simulink model "Satellite_Design_Model_2019ver"  (R2019a)
settings: Solver=ode45  StartTime=0.0  StopTime=500  RelTol=1e-3
undefined symbols (not defined in the file or in its folder): km, s, sigbuilder_block
libraries: simulink_extras x10, sharedtransform x7, simulink x1, aerolibcelestial x1
settings Model: Creator=MSI  LastModifiedBy=MSI
settings SolverCC: ZeroCrossAlgorithm=Adaptive
settings OptimizationCC: LifeSpan=inf
settings DebuggingCC: IgnoredZcDiagnostic=none  SFExecutionAtInitializationDiag=none  ArithmeticOperatorsInVariantConditions=warning
settings HardwareCC: ProdBitPerSizeT=32  ProdBitPerPtrDiffT=32  ProdWordSize=32  ProdHWDeviceType=Specified
settings CodeAppCC: StateflowObjectComments=on

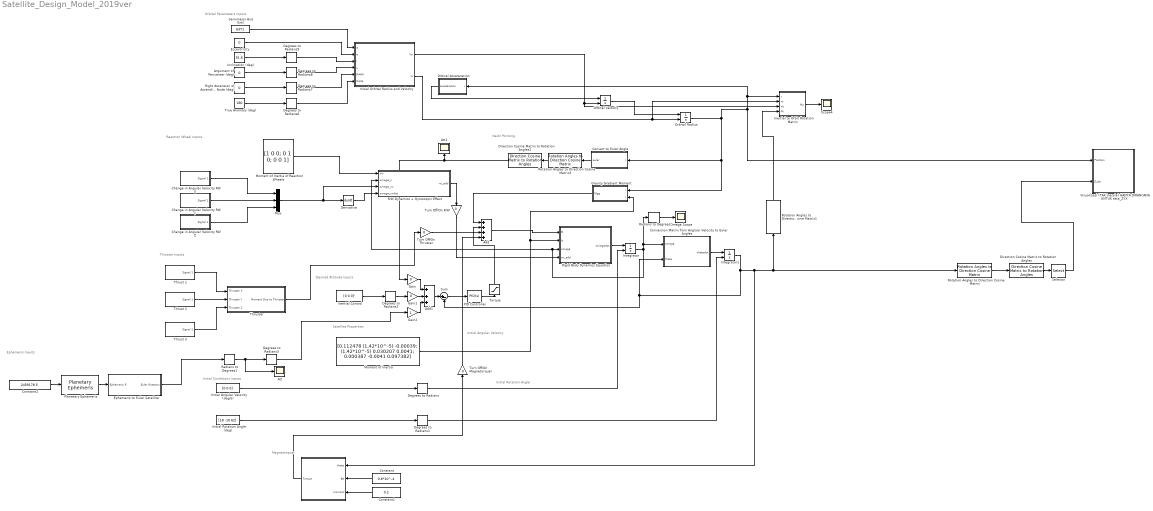
== system Satellite_Design_Model_2019ver ==
  note: Nadir Pointing
  note: Ephemeris Inputs
  note: Magnetorquer
  note: Initial Conditions Inputs
  note: Satellite Properties
  note: Desired Attitude Inputs
  note: Orbital Parameters Inputs
  note: Thruster Inputs
  note: Reaction Wheel Inputs
  note: Initial Rotation Angle
  note: Initial Angular Velocity
  " " : MATLAB Function  TreatAsAtomicUnit=on
  Add : Sum  Inputs=++++
  Add1 : Sum  Inputs=+++
  Argument of Pericenter (deg) : Constant  Value=0
  Att : Scope
  Att1 : Scope
  Change in Angular Velocity RW X : Subsystem  Tag=STV Subsys  LoadFcn=sigbuilder_block('load');  StartFcn=sigbuilder_block('start');  StopFcn=sigbuilder_block('stop');  ClipboardFcn=sigbuilder_block('clipboard');  mask(Sigbuilder block){tuvar=[0:10]}
      mask help: Simulink:masks:SigbuilderBlock_MD
      mask init:
      | if ~strcmp(get_param(bdroot(gcbh),'SimulationStatus'),'stopped') tuvar = sigbuilder_block('maskInit'); end
      settings: CopyFcn=sigbuilder_block('copy');  DeleteFcn=sigbuilder_block('delete');  ModelCloseFcn=sigbuilder_block('modelClose');  PreSaveFcn=sigbuilder_block('preSave');  PauseFcn=sigbuilder_block('pause');  ContinueFcn=sigbuilder_block('continue');  NameChangeFcn=sigbuilder_block('namechange');  OpenFcn=sigbuilder_block('open',[63.6 87.6 1024.8 449.4 ]);  CloseFcn=sigbuilder_block('close');
      mask Display: plot(0, 0, 100, 100,[2, 2, 32, 32, 2], [68, 8, 8, 68, 68],[32, 2], [38, 38], [32, 19, 2],[53, 60, 44], [32, 17, 17, 2],[16, 16, 31, 31]);txt = getActiveGroup(gcbh);text(2, 100, txt,'verticalAlignment', 'top');
  Change in Angular Velocity RW Y : Subsystem  Tag=STV Subsys  LoadFcn=sigbuilder_block('load');  StartFcn=sigbuilder_block('start');  StopFcn=sigbuilder_block('stop');  ClipboardFcn=sigbuilder_block('clipboard');  mask(Sigbuilder block){tuvar=[0:10]}
      mask help: Simulink:masks:SigbuilderBlock_MD
      mask init:
      | if ~strcmp(get_param(bdroot(gcbh),'SimulationStatus'),'stopped') tuvar = sigbuilder_block('maskInit'); end
      settings: CopyFcn=sigbuilder_block('copy');  DeleteFcn=sigbuilder_block('delete');  ModelCloseFcn=sigbuilder_block('modelClose');  PreSaveFcn=sigbuilder_block('preSave');  PauseFcn=sigbuilder_block('pause');  ContinueFcn=sigbuilder_block('continue');  NameChangeFcn=sigbuilder_block('namechange');  OpenFcn=sigbuilder_block('open',[0 30 1024.5 488.25 ]);  CloseFcn=sigbuilder_block('close');
      mask Display: plot(0, 0, 100, 100,[2, 2, 32, 32, 2], [68, 8, 8, 68, 68],[32, 2], [38, 38], [32, 19, 2],[53, 60, 44], [32, 17, 17, 2],[16, 16, 31, 31]);txt = getActiveGroup(gcbh);text(2, 100, txt,'verticalAlignment', 'top');
  Change in Angular Velocity RW Z : Subsystem  Tag=STV Subsys  LoadFcn=sigbuilder_block('load');  StartFcn=sigbuilder_block('start');  StopFcn=sigbuilder_block('stop');  ClipboardFcn=sigbuilder_block('clipboard');  mask(Sigbuilder block){tuvar=[0:10]}
      mask help: Simulink:masks:SigbuilderBlock_MD
      mask init:
      | if ~strcmp(get_param(bdroot(gcbh),'SimulationStatus'),'stopped') tuvar = sigbuilder_block('maskInit'); end
      settings: CopyFcn=sigbuilder_block('copy');  DeleteFcn=sigbuilder_block('delete');  ModelCloseFcn=sigbuilder_block('modelClose');  PreSaveFcn=sigbuilder_block('preSave');  PauseFcn=sigbuilder_block('pause');  ContinueFcn=sigbuilder_block('continue');  NameChangeFcn=sigbuilder_block('namechange');  OpenFcn=sigbuilder_block('open',[93.6 105.6 928.8 430.2 ]);  CloseFcn=sigbuilder_block('close');
      mask Display: plot(0, 0, 100, 100,[2, 2, 32, 32, 2], [68, 8, 8, 68, 68],[32, 2], [38, 38], [32, 19, 2],[53, 60, 44], [32, 17, 17, 2],[16, 16, 31, 31]);txt = getActiveGroup(gcbh);text(2, 100, txt,'verticalAlignment', 'top');
  Constant : Constant  Value=0.6*10^-4
  Constant1 : Constant  Value=0.2
  Constant2 : Constant  Value=2459178.5
  Conversion Matrix from Angluar Velocity to Euler Angles : MATLAB Function  TreatAsAtomicUnit=on
  Convert to Euler Angle : MATLAB Function  TreatAsAtomicUnit=on
  Degrees to Radians{,1..3,6..9} (8 alike) : simulink_extras/Transformations/Degrees to Radians
  Derivative : Derivative
  Direction Cosine Matrix to Rotation Angles : sharedtransform/Direction Cosine Matrix to Rotation Angles  rotationOrder=ZYX  aMode=aMode  action=None  tolerance=eps(2)
      settings: SourceProductBaseCode=AE,PW,MT,UV,VE,VP
  Direction Cosine Matrix to Rotation Angles2 : sharedtransform/Direction Cosine Matrix to Rotation Angles  rotationOrder=XYZ  aMode=aMode  action=None  tolerance=eps(2)
      settings: SourceProductName=Aerospace Blockset  SourceProductBaseCode=AE
  Eccentricity : Constant  Value=0
  Ephemeris to Euler Satellite : Subsystem
  Gain : Gain  Gain=0
  Gain1 : Gain  Gain=0
  Gain2 : Gain
  Gravity Gradient Moment : Subsystem
  Inclination (deg) : Constant  Value=51.6
  Inertial Control : Constant  Value=[0 0 0]'
  Inertial to Orbit Rotation Matrix : MATLAB Function  TreatAsAtomicUnit=on
  Initial Angular Velocity (deg/s) : Constant  Value=[0 0 0]
  Initial Orbital Radius and Velocity : MATLAB Function  TreatAsAtomicUnit=on
  Initial Rotation Angle (deg) : Constant  Value=[18 -10 62]
  Integrator : Integrator  InitialConditionSource=external
  Integrator1 : Integrator  InitialConditionSource=external
  Moment of Inertia : Constant  Value=[0.112478 (1.42*10^-5) -0.00039; (1.42*10^-5) 0.030207 0.0041; 0.000387 -0.0041 0.097382]
  Moment of Inertia of Reaction Wheels : Constant  Value=[1 0 0; 0 1 0; 0 0 1]
  Mux : Mux  Inputs=3
  Omega Scope : Scope
  Orbital Acceleration : MATLAB Function  TreatAsAtomicUnit=on
  Orbital Radius : Integrator  InitialConditionSource=external
  Orbital Velocity : Integrator  InitialConditionSource=external
  PID Controller : simulink/Continuous/PID Controller  Controller=PID  Form=Parallel  TimeDomain=Continuous-time  SampleTime=-1  IntegratorMethod=Forward Euler  FilterMethod=Forward Euler  ControllerParametersSource=internal  P=2  I=0  D=20  UseFilter=on  N=100  TunerSelectOption=Transfer Function Based (PID Tuner App)  InitialConditionSource=internal  InitialConditionForIntegrator=0  InitialConditionForFilter=0  DifferentiatorICPrevScaledInput=0  ExternalReset=none  TrackingMode=off  Kt=1  LimitOutput=off  UpperSaturationLimit=inf  LowerSaturationLimit=-inf  LinearizeAsGain=on  AntiWindupMode=none  Kb=1  POutMin=[]  POutMax=[]  IOutMin=[]  IOutMax=[]  DOutMin=[]  DOutMax=[]  NOutMin=[]  NOutMax=[]  SumOutMin=[]  SumOutMax=[]  SaturationOutMin=[]  SaturationOutMax=[]  PParamMin=[]  PParamMax=[]  IParamMin=[]  IParamMax=[]  DParamMin=[]  DParamMax=[]  NParamMin=[]  NParamMax=[]  KbParamMin=[]  KbParamMax=[]  KtParamMin=[]  KtParamMax=[]  KbOutMin=[]  KbOutMax=[]  KtOutMin=[]  KtOutMax=[]  IntegratorOutMin=[]  IntegratorOutMax=[]  FilterOutMin=[]  FilterOutMax=[]  SumI1OutMin=[]  SumI1OutMax=[]  SumI2OutMin=[]  SumI2OutMax=[]  SumI3OutMin=[]  SumI3OutMax=[]  SumI4OutMin=[]  SumI4OutMax=[]  SumDOutMin=[]  SumDOutMax=[]  DifferentiatorOutMin=[]  DifferentiatorOutMax=[]  FilterDiffOutCoefMin=[]  FilterDiffOutCoefMax=[]  ReciprocalOutMin=[]  ReciprocalOutMax=[]  SumDenOutMin=[]  SumDenOutMax=[]  SumNumOutMin=[]  SumNumOutMax=[]  DivideOutMin=[]  DivideOutMax=[]  IntegratorContinuousStateAttributes=''  IntegratorStateMustResolveToSignalObject=off  IntegratorRTWStateStorageClass=Auto  FilterContinuousStateAttributes=''  FilterStateMustResolveToSignalObject=off  FilterRTWStateStorageClass=Auto  ParallelPVariant=InternalParameters  IdealPVariant=Disabled  IVariant=InternalParameters  DVariant=InternalParameters  IntegratorVariant=Continuous  SatVariant=Disabled  AWVariant=Passthrough  PCopyVariant=Disabled  TRVariant=Disabled  FdbkBlocksVariant=Forward  IdealPFdbkVariant=Disabled  SatFdbkVariant=Disabled  DerivativeFilterVariant=ContFilter  NVariant=InternalParameters  NCopyVariant=Disabled  FilterICVariant=InternalICsFilter  IntegratorICVariant=InternalICs  ExternalResetVariant=Disabled  TRSumVariant=Passthrough  SumFdbkVariant=Disabled  SumVariant=Sum_PID
  Planetary Ephemeris : aerolibcelestial/Planetary Ephemeris  kmflag=km,km/s  epochflag=Julian date  de=DE405  nCenter=Earth  nTarget=Neptune  errorflag=Error  velflag=off
      settings: SourceProductName=Aerospace Blockset  SourceProductBaseCode=AE
  R/W Dynamics + Gyroscopic Effect : MATLAB Function  TreatAsAtomicUnit=on
  Radians to Degrees : simulink_extras/Transformations/Radians to Degrees
  Radians to Degrees1 : simulink_extras/Transformations/Radians to Degrees
  Right Ascension of Ascending Node (deg) : Constant  Value=0
  "Rigid Body Dynamics Equation " : MATLAB Function  TreatAsAtomicUnit=on
  Rotation Angles to Direction Cosine Matrix : sharedtransform/Rotation Angles to Direction Cosine Matrix  rotationOrder=XYZ  aMode=aMode
      settings: SourceProductBaseCode=AE,PW,MT,UV,VE,VP
  Rotation Angles to Direction Cosine Matrix1 : sharedtransform/Rotation Angles to Direction Cosine Matrix  rotationOrder=XYZ  aMode=aMode
      settings: SourceProductBaseCode=AE,PW,MT,UV,VE,VP
  Rotation Angles to Direction Cosine Matrix3 : sharedtransform/Rotation Angles to Direction Cosine Matrix  rotationOrder=ZYX  aMode=aMode
      settings: SourceProductBaseCode=AE
  Scope4 : Scope
  Selector : Selector  InputPortWidth=3  IndexOptions=Index vector (dialog)  Indices=[3 2 1]  OutputSizes=1
  Semimajor Axis (km) : Constant  Value=6371
  Sum : Sum  Inputs=|+-
  Thrust 1 : Subsystem  Tag=STV Subsys  LoadFcn=sigbuilder_block('load');  StartFcn=sigbuilder_block('start');  StopFcn=sigbuilder_block('stop');  ClipboardFcn=sigbuilder_block('clipboard');  mask(Sigbuilder block){tuvar=[0:10]}
      mask help: Simulink:masks:SigbuilderBlock_MD
      mask init:
      | if ~strcmp(get_param(bdroot(gcbh),'SimulationStatus'),'stopped') tuvar = sigbuilder_block('maskInit'); end
      settings: CopyFcn=sigbuilder_block('copy');  DeleteFcn=sigbuilder_block('delete');  ModelCloseFcn=sigbuilder_block('modelClose');  PreSaveFcn=sigbuilder_block('preSave');  PauseFcn=sigbuilder_block('pause');  ContinueFcn=sigbuilder_block('continue');  NameChangeFcn=sigbuilder_block('namechange');  OpenFcn=sigbuilder_block('open',[121.8 6 1024.8 449.4 ]);  CloseFcn=sigbuilder_block('close');
      mask Display: plot(0, 0, 100, 100,[2, 2, 32, 32, 2], [68, 8, 8, 68, 68],[32, 2], [38, 38], [32, 19, 2],[53, 60, 44], [32, 17, 17, 2],[16, 16, 31, 31]);txt = getActiveGroup(gcbh);text(2, 100, txt,'verticalAlignment', 'top');
  Thrust 2 : Subsystem  Tag=STV Subsys  LoadFcn=sigbuilder_block('load');  StartFcn=sigbuilder_block('start');  StopFcn=sigbuilder_block('stop');  ClipboardFcn=sigbuilder_block('clipboard');  mask(Sigbuilder block){tuvar=[0:10]}
      mask help: Simulink:masks:SigbuilderBlock_MD
      mask init:
      | if ~strcmp(get_param(bdroot(gcbh),'SimulationStatus'),'stopped') tuvar = sigbuilder_block('maskInit'); end
      settings: CopyFcn=sigbuilder_block('copy');  DeleteFcn=sigbuilder_block('delete');  ModelCloseFcn=sigbuilder_block('modelClose');  PreSaveFcn=sigbuilder_block('preSave');  PauseFcn=sigbuilder_block('pause');  ContinueFcn=sigbuilder_block('continue');  NameChangeFcn=sigbuilder_block('namechange');  OpenFcn=sigbuilder_block('open',[0 30 1024.5 488.25 ]);  CloseFcn=sigbuilder_block('close');
      mask Display: plot(0, 0, 100, 100,[2, 2, 32, 32, 2], [68, 8, 8, 68, 68],[32, 2], [38, 38], [32, 19, 2],[53, 60, 44], [32, 17, 17, 2],[16, 16, 31, 31]);txt = getActiveGroup(gcbh);text(2, 100, txt,'verticalAlignment', 'top');
  Thrust 3 : Subsystem  Tag=STV Subsys  LoadFcn=sigbuilder_block('load');  StartFcn=sigbuilder_block('start');  StopFcn=sigbuilder_block('stop');  ClipboardFcn=sigbuilder_block('clipboard');  mask(Sigbuilder block){tuvar=[0:10]}
      mask help: Simulink:masks:SigbuilderBlock_MD
      mask init:
      | if ~strcmp(get_param(bdroot(gcbh),'SimulationStatus'),'stopped') tuvar = sigbuilder_block('maskInit'); end
      settings: CopyFcn=sigbuilder_block('copy');  DeleteFcn=sigbuilder_block('delete');  ModelCloseFcn=sigbuilder_block('modelClose');  PreSaveFcn=sigbuilder_block('preSave');  PauseFcn=sigbuilder_block('pause');  ContinueFcn=sigbuilder_block('continue');  NameChangeFcn=sigbuilder_block('namechange');  OpenFcn=sigbuilder_block('open',[93.6 105.6 928.8 430.2 ]);  CloseFcn=sigbuilder_block('close');
      mask Display: plot(0, 0, 100, 100,[2, 2, 32, 32, 2], [68, 8, 8, 68, 68],[32, 2], [38, 38], [32, 19, 2],[53, 60, 44], [32, 17, 17, 2],[16, 16, 31, 31]);txt = getActiveGroup(gcbh);text(2, 100, txt,'verticalAlignment', 'top');
  Thruster : Subsystem
  Torque : Saturate  UpperLimit=0.00635  LowerLimit=-0.00635
  True Anomaly (deg) : Constant  Value=180
  Turn Off/On Magnetorquer : Gain  Gain=0
  Turn Off/On R/W : Gain  Gain=0
  Turn Off/On Thruster : Gain  Gain=0
  Visualisasi (TAK Inersia) HANYA DIRANCANG UNTUK teta_ZYX : Subsystem  mask(6DoF_Animation){u1=[-20000 20000 -20000 20000 -20000 20000], u2=1, u3=5000, u4=[0 0 0], u5=Fixed Position, u6=[40000 20000 30000], u7=30, u8=on}
      mask prompts: u1 "Axes limits [xmin xmax ymin ymax zmin zmax]:"; u2 "Time interval between updates:"; u3 "Size of craft displayed:"; u4 "Static object position [xp yp zp]:"; u5 "Enter view:"; u6 "Position of camera [xc yc zc]:"; u7 "View angle:"; u8 "Enable animation"
      mask init:
      | Config.axes = u1;
      | Config.update = u2;
      | Config.craft = u3;
      | Config.target = u4;
      | Config.camera_view = u5;
      | Config.camera_pos = u6;
      | Config.view = u7;
      | Config.Animenable = u8;
      | Config.Model = bdroot(gcb);
      mask TypeOptions u5: Fixed Position | Cockpit | Fly alongside
      mask Display:
      | port_label('input',1,'x_e','texmode','on');
      | port_label('input',2,'\phi \theta \psi','texmode','on');
      | [xp yp] = aeroimage('anim',gcbh);
      | patch(xp,yp)
  wires:
  Selector/1 -> Visualisasi (TAK Inersia) HANYA DIRANCANG UNTUK teta_ZYX/2(Euler)
  Direction Cosine Matrix to Rotation Angles/1 -> Selector/1
  Rotation Angles to Direction Cosine Matrix/1 -> Direction Cosine Matrix to Rotation Angles/1
  Integrator/1 -> Radians to Degrees/1, Conversion Matrix from Angluar Velocity to Euler Angles/1(omega), R/W Dynamics + Gyroscopic Effect/2(omega_s), "Rigid Body Dynamics Equation "/3(omega)
  Conversion Matrix from Angluar Velocity to Euler Angles/1(thetadot) -> Integrator1/1
  Degrees to Radians/1 -> Integrator/2
  Degrees to Radians1/1 -> Integrator1/2
  Initial Angular Velocity (deg/s)/1 -> Degrees to Radians/1
  Integrator1/1 -> Sum/2, Conversion Matrix from Angluar Velocity to Euler Angles/2(theta), Rotation Angles to Direction Cosine Matrix/1, Rotation Angles to Direction Cosine Matrix1/1, " "/1(theta)
  Radians to Degrees/1 -> Omega Scope/1
  Moment of Inertia/1 -> Gravity Gradient Moment/2(I), "Rigid Body Dynamics Equation "/2(Is)
  Degrees to Radians9/1 -> Initial Orbital Radius and Velocity/3(i)
  Eccentricity/1 -> Initial Orbital Radius and Velocity/2(e)
  Inertial to Orbit Rotation Matrix/1(Mo) -> Scope4/1
  Rotation Angles to Direction Cosine Matrix1/1 -> Inertial to Orbit Rotation Matrix/4(Mi)
  Initial Orbital Radius and Velocity/1(Vo) -> Inertial to Orbit Rotation Matrix/3(Vo), Orbital Velocity/2
  Degrees to Radians6/1 -> Initial Orbital Radius and Velocity/6(theta)
  Degrees to Radians8/1 -> Initial Orbital Radius and Velocity/4(u)
  Degrees to Radians7/1 -> Initial Orbital Radius and Velocity/5(RAAN)
  Initial Orbital Radius and Velocity/2(ro) -> Inertial to Orbit Rotation Matrix/2(ro), Orbital Radius/2
  Argument of Pericenter (deg)/1 -> Degrees to Radians8/1
  Right Ascension of Ascending Node (deg)/1 -> Degrees to Radians7/1
  Orbital Acceleration/1(acceleration) -> Orbital Velocity/1
  Inclination (deg)/1 -> Degrees to Radians9/1
  Orbital Velocity/1 -> Orbital Radius/1
  Semimajor Axis (km)/1 -> Initial Orbital Radius and Velocity/1(a)
  True Anomaly (deg)/1 -> Degrees to Radians6/1
  Thrust 1/1(Signal 1) -> Thruster/1(Thruster X)
  Thrust 2/1(Signal 1) -> Thruster/2(Thruster Y)
  Thrust 3/1(Signal 1) -> Thruster/3(Thruster Z)
  Gravity Gradient Moment/1(Mgg) -> Add/1
  Sum/1 -> PID Controller/1
  PID Controller/1 -> Torque/1
  Add/1 -> "Rigid Body Dynamics Equation "/1(M)
  Torque/1 -> Add/2
  Thruster/1(Moment Due to Thruster) -> Turn Off/On Thruster/1
  Change in Angular Velocity RW X/1(Signal 1) -> Mux/1
  Change in Angular Velocity RW Y/1(Signal 1) -> Mux/2
  Change in Angular Velocity RW Z/1(Signal 1) -> Mux/3
  "Rigid Body Dynamics Equation "/1(omegadot) -> Integrator/1
  Moment of Inertia of Reaction Wheels/1 -> R/W Dynamics + Gyroscopic Effect/1(Irw)
  Mux/1 -> Derivative/1, R/W Dynamics + Gyroscopic Effect/3(omega_rw)
  Derivative/1 -> R/W Dynamics + Gyroscopic Effect/4(omega_rwdot)
  R/W Dynamics + Gyroscopic Effect/1(rw_add) -> Turn Off/On R/W/1
  Turn Off/On R/W/1 -> "Rigid Body Dynamics Equation "/4(rw_add)
  Constant/1 -> " "/2(Be)
  Constant1/1 -> " "/3(moment)
  " "/1(Torque) -> Turn Off/On Magnetorquer/1
  Turn Off/On Magnetorquer/1 -> Add/4
  Turn Off/On Thruster/1 -> Add/3
  Inertial Control/1 -> Degrees to Radians2/1
  Constant2/1 -> Planetary Ephemeris/1
  Orbital Radius/1 -> Gravity Gradient Moment/1(r), Convert to Euler Angle/1(r), Visualisasi (TAK Inersia) HANYA DIRANCANG UNTUK teta_ZYX/1(Position), Inertial to Orbit Rotation Matrix/1(r), Orbital Acceleration/1(r)
  Rotation Angles to Direction Cosine Matrix3/1 -> Direction Cosine Matrix to Rotation Angles2/1
  Convert to Euler Angle/1(euler) -> Rotation Angles to Direction Cosine Matrix3/1
  Direction Cosine Matrix to Rotation Angles2/1 -> Att1/1, Gain/1
  Planetary Ephemeris/1 -> Ephemeris to Euler Satellite/1(Ephemeris R)
  Add1/1 -> Sum/1
  Degrees to Radians2/1 -> Gain1/1
  Gain/1 -> Add1/1
  Gain1/1 -> Add1/2
  Gain2/1 -> Add1/3
  Ephemeris to Euler Satellite/1(Euler Rotation) -> Radians to Degrees1/1
  Initial Rotation Angle (deg)/1 -> Degrees to Radians1/1
  Degrees to Radians3/1 -> Gain2/1
  Radians to Degrees1/1 -> Att/1, Degrees to Radians3/1

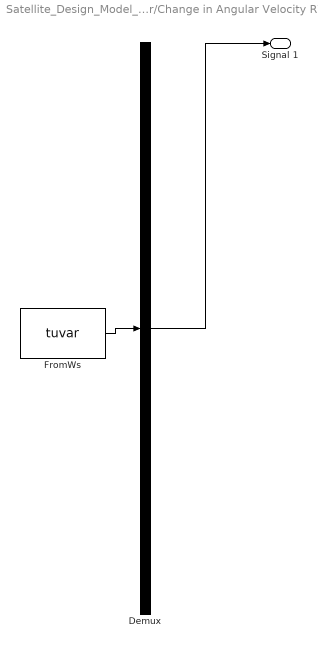
== system Satellite_Design_Model_2019ver/Change in Angular Velocity RW X ==
  Demux : Demux  Tag=STV Demux  Outputs=1
  FromWs : FromWorkspace  Tag=STV FromWs  VariableName=tuvar  SampleTime=0
      SigBuilderData=|
      | common.afterFinalStr = 'Extrapolate'
      | common.sampleTime = 0
      | dataSet.timeRange = [0 100]
      | dataSet.name = 'Group 1'
      | sbobj.Groups.Name = 'Group 1'
      | sbobj.Groups.Signals.Name = 'Signal 1'
      | sbobj.Groups.Signals.XData = [0 14.4 14.4 36.9 70.4 90.1 100]
      | sbobj.Groups.Signals.YData = [0.195 0.195 0 0 0 0 0]
      | sbobj.Groups.TimeRange = [0 100]
  Signal 1 : Outport  Tag=STV Outport  VectorParamsAs1DForOutWhenUnconnected=on
  wires:
  Demux/1 -> Signal 1/1
  FromWs/1 -> Demux/1

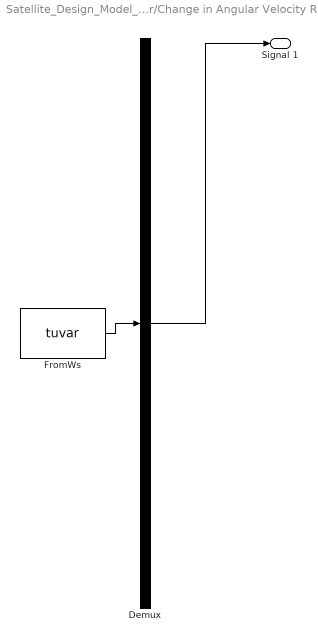
== system Satellite_Design_Model_2019ver/Change in Angular Velocity RW Y ==
  Demux : Demux  Tag=STV Demux  Outputs=1
  FromWs : FromWorkspace  Tag=STV FromWs  VariableName=tuvar  SampleTime=0
      SigBuilderData=|
      | common.afterFinalStr = 'Extrapolate'
      | common.sampleTime = 0
      | dataSet.timeRange = [0 100]
      | dataSet.name = 'Group 1'
      | sbobj.Groups.Name = 'Group 1'
      | sbobj.Groups.Signals.Name = 'Signal 1'
      | sbobj.Groups.Signals.XData = [0 40 52 100]
      | sbobj.Groups.Signals.YData = [0 0 0 0]
      | sbobj.Groups.TimeRange = [0 100]
  Signal 1 : Outport  Tag=STV Outport  VectorParamsAs1DForOutWhenUnconnected=on
  wires:
  FromWs/1 -> Demux/1
  Demux/1 -> Signal 1/1

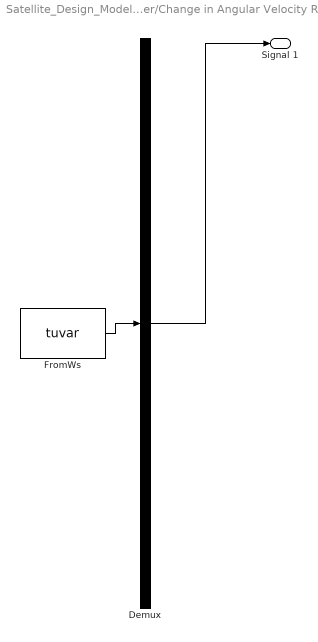
== system Satellite_Design_Model_2019ver/Change in Angular Velocity RW Z ==
  Demux : Demux  Tag=STV Demux  Outputs=1
  FromWs : FromWorkspace  Tag=STV FromWs  VariableName=tuvar  SampleTime=0
      SigBuilderData=|
      | common.afterFinalStr = 'Extrapolate'
      | common.sampleTime = 0
      | dataSet.timeRange = [0 100]
      | dataSet.name = 'Group 1'
      | sbobj.Groups.Name = 'Group 1'
      | sbobj.Groups.Signals.Name = 'Signal 1'
      | sbobj.Groups.Signals.XData = [0 80 90 100]
      | sbobj.Groups.Signals.YData = [0 0 0 0]
      | sbobj.Groups.TimeRange = [0 100]
  Signal 1 : Outport  Tag=STV Outport  VectorParamsAs1DForOutWhenUnconnected=on
  wires:
  Demux/1 -> Signal 1/1
  FromWs/1 -> Demux/1

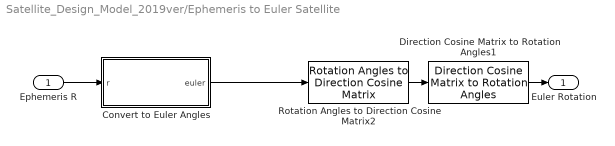
== system Satellite_Design_Model_2019ver/Ephemeris to Euler Satellite ==
  Ephemeris R : Inport
  Convert to Euler Angles : MATLAB Function  TreatAsAtomicUnit=on
  Direction Cosine Matrix to Rotation Angles1 : sharedtransform/Direction Cosine Matrix to Rotation Angles  rotationOrder=XYZ  aMode=aMode  action=None  tolerance=eps(2)
      settings: SourceProductName=Aerospace Blockset  SourceProductBaseCode=AE
  Rotation Angles to Direction Cosine Matrix2 : sharedtransform/Rotation Angles to Direction Cosine Matrix  rotationOrder=ZYX  aMode=aMode
      settings: SourceProductBaseCode=AE
  Euler Rotation : Outport
  wires:
  Direction Cosine Matrix to Rotation Angles1/1 -> Euler Rotation/1
  Rotation Angles to Direction Cosine Matrix2/1 -> Direction Cosine Matrix to Rotation Angles1/1
  Convert to Euler Angles/1(euler) -> Rotation Angles to Direction Cosine Matrix2/1
  Ephemeris R/1 -> Convert to Euler Angles/1(r)

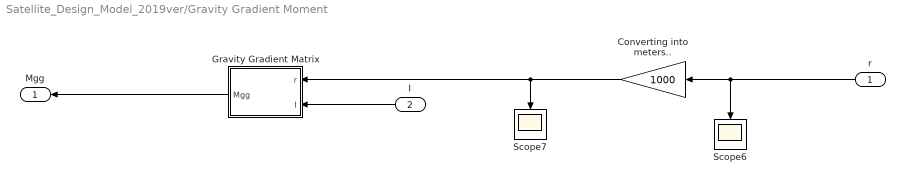
== system Satellite_Design_Model_2019ver/Gravity Gradient Moment ==
  r : Inport
  I : Inport  Port=2
  Converting into meters.. : Gain  Gain=1000
  Gravity Gradient Matrix : MATLAB Function  TreatAsAtomicUnit=on
  Scope6 : Scope
  Scope7 : Scope
  Mgg : Outport  VectorParamsAs1DForOutWhenUnconnected=on
  wires:
  Converting into meters../1 -> Gravity Gradient Matrix/1(r), Scope7/1
  I/1 -> Gravity Gradient Matrix/2(I)
  Gravity Gradient Matrix/1(Mgg) -> Mgg/1
  r/1 -> Scope6/1, Converting into meters../1

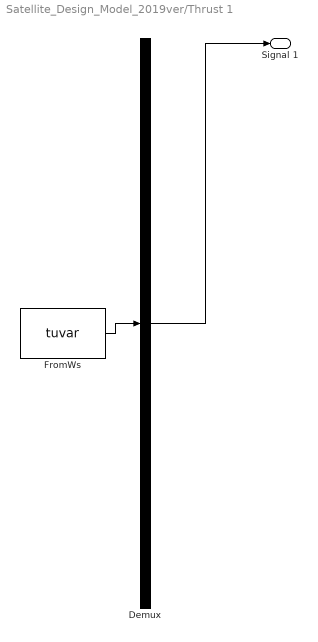
== system Satellite_Design_Model_2019ver/Thrust 1 ==
  Demux : Demux  Tag=STV Demux  Outputs=1
  FromWs : FromWorkspace  Tag=STV FromWs  VariableName=tuvar  SampleTime=0
      SigBuilderData=|
      | common.afterFinalStr = 'Extrapolate'
      | common.sampleTime = 0
      | dataSet.timeRange = [0 100]
      | dataSet.name = 'Group 1'
      | sbobj.Groups.Name = 'Group 1'
      | sbobj.Groups.Signals.Name = 'Signal 1'
      | sbobj.Groups.Signals.XData = [0 14.4 14.4 36.9 36.9 70.4 70.4 90.1 90.1 100]
      | sbobj.Groups.Signals.YData = [0 0 -0.124 -0.124 0 0 0.075 0.075 0 0]
      | sbobj.Groups.TimeRange = [0 100]
  Signal 1 : Outport  Tag=STV Outport  VectorParamsAs1DForOutWhenUnconnected=on
  wires:
  Demux/1 -> Signal 1/1
  FromWs/1 -> Demux/1

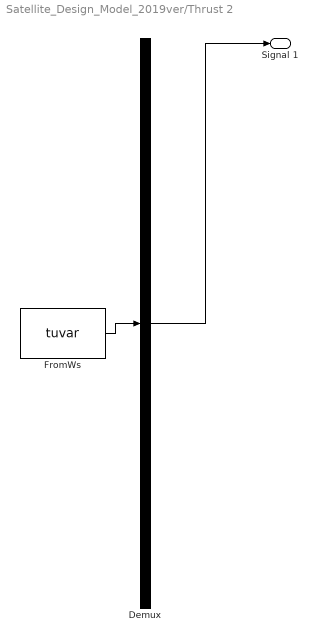
== system Satellite_Design_Model_2019ver/Thrust 2 ==
  Demux : Demux  Tag=STV Demux  Outputs=1
  FromWs : FromWorkspace  Tag=STV FromWs  VariableName=tuvar  SampleTime=0
      SigBuilderData=|
      | common.afterFinalStr = 'Extrapolate'
      | common.sampleTime = 0
      | dataSet.timeRange = [0 100]
      | dataSet.name = 'Group 1'
      | sbobj.Groups.Name = 'Group 1'
      | sbobj.Groups.Signals.Name = 'Signal 1'
      | sbobj.Groups.Signals.XData = [0 40 40 52 52 100]
      | sbobj.Groups.Signals.YData = [0.5 0.5 -0.18 -0.18 0 0]
      | sbobj.Groups.TimeRange = [0 100]
  Signal 1 : Outport  Tag=STV Outport  VectorParamsAs1DForOutWhenUnconnected=on
  wires:
  FromWs/1 -> Demux/1
  Demux/1 -> Signal 1/1

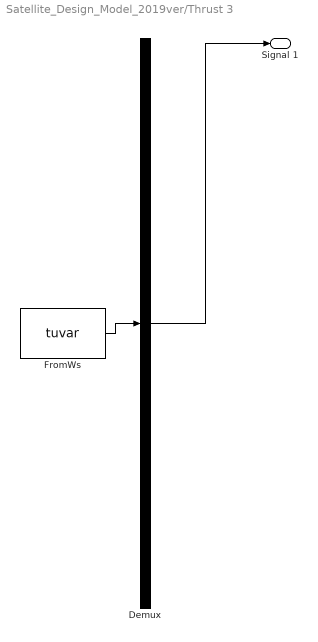
== system Satellite_Design_Model_2019ver/Thrust 3 ==
  Demux : Demux  Tag=STV Demux  Outputs=1
  FromWs : FromWorkspace  Tag=STV FromWs  VariableName=tuvar  SampleTime=0
      SigBuilderData=|
      | common.afterFinalStr = 'Extrapolate'
      | common.sampleTime = 0
      | dataSet.timeRange = [0 100]
      | dataSet.name = 'Group 1'
      | sbobj.Groups.Name = 'Group 1'
      | sbobj.Groups.Signals.Name = 'Signal 1'
      | sbobj.Groups.Signals.XData = [0 80 80 90 90 100]
      | sbobj.Groups.Signals.YData = [0 0 -0.0349 -0.0349 0 0]
      | sbobj.Groups.TimeRange = [0 100]
  Signal 1 : Outport  Tag=STV Outport  VectorParamsAs1DForOutWhenUnconnected=on
  wires:
  Demux/1 -> Signal 1/1
  FromWs/1 -> Demux/1

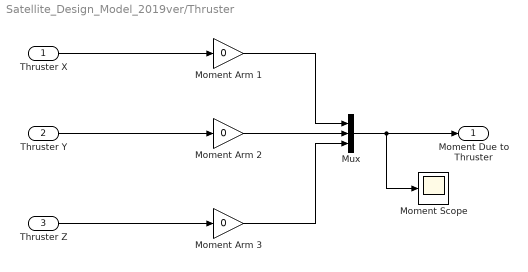
== system Satellite_Design_Model_2019ver/Thruster ==
  Thruster X : Inport
  Thruster Y : Inport  Port=2
  Thruster Z : Inport  Port=3
  Moment Arm 1 : Gain  Gain=0
  Moment Arm 2 : Gain  Gain=0
  Moment Arm 3 : Gain  Gain=0
  Moment Scope : Scope
  Mux : Mux  Inputs=3
  Moment Due to Thruster : Outport  VectorParamsAs1DForOutWhenUnconnected=on
  wires:
  Thruster Y/1 -> Moment Arm 2/1
  Thruster X/1 -> Moment Arm 1/1
  Moment Arm 2/1 -> Mux/2
  Moment Arm 3/1 -> Mux/3
  Thruster Z/1 -> Moment Arm 3/1
  Moment Arm 1/1 -> Mux/1
  Mux/1 -> Moment Due to Thruster/1, Moment Scope/1

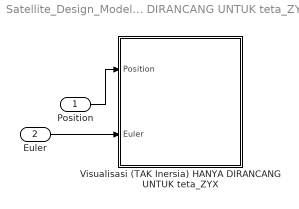
== system Satellite_Design_Model_2019ver/Visualisasi (TAK Inersia) HANYA DIRANCANG UNTUK teta_ZYX ==
  Position : Inport
  Euler : Inport  Port=2
  Visualisasi (TAK Inersia) HANYA DIRANCANG UNTUK teta_ZYX : Subsystem  mask(6DoF_Animation){u1=[-20000 20000 -20000 20000 -20000 20000], u2=1, u3=5000, u4=[0 0 0], u5=Fixed Position, u6=[40000 20000 30000], u7=30, u8=on}
      mask prompts: u1 "Axes limits [xmin xmax ymin ymax zmin zmax]:"; u2 "Time interval between updates:"; u3 "Size of craft displayed:"; u4 "Static object position [xp yp zp]:"; u5 "Enter view:"; u6 "Position of camera [xc yc zc]:"; u7 "View angle:"; u8 "Enable animation"
      mask init:
      | Config.axes = u1;
      | Config.update = u2;
      | Config.craft = u3;
      | Config.target = u4;
      | Config.camera_view = u5;
      | Config.camera_pos = u6;
      | Config.view = u7;
      | Config.Animenable = u8;
      | Config.Model = bdroot(gcb);
      mask TypeOptions u5: Fixed Position | Cockpit | Fly alongside
      mask Display:
      | port_label('input',1,'x_e','texmode','on');
      | port_label('input',2,'\phi \theta \psi','texmode','on');
      | [xp yp] = aeroimage('anim',gcbh);
      | patch(xp,yp)
  wires:
  Position/1 -> Visualisasi (TAK Inersia) HANYA DIRANCANG UNTUK teta_ZYX/1(Position)
  Euler/1 -> Visualisasi (TAK Inersia) HANYA DIRANCANG UNTUK teta_ZYX/2(Euler)

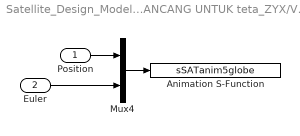
== system Satellite_Design_Model_2019ver/Visualisasi (TAK Inersia) HANYA DIRANCANG UNTUK teta_ZYX/Visualisasi (TAK Inersia) HANYA DIRANCANG UNTUK teta_ZYX ==
  Position : Inport
  Euler : Inport  Port=2
  Animation S-Function : S-Function  FunctionName=sSATanim5globe  Parameters=Config  SFunctionDeploymentMode=off  EnableBusSupport=off
  Mux4 : Mux  Inputs=2
  wires:
  Position/1 -> Mux4/1
  Mux4/1 -> Animation S-Function/1
  Euler/1 -> Mux4/2

== matlab function Satellite_Design_Model_2019ver/Orbital Acceleration ==
  data: r input; acceleration output
function acceleration = fcn(r)
miu =3.986E5; 

acceleration = [-miu*r(1)/(norm(r))^3 -miu*r(2)/(norm(r))^3 -miu*r(3)/(norm(r))^3];

== matlab function Satellite_Design_Model_2019ver/Rigid Body Dynamics Equation  ==
  data: M input; Is input; omega input; omegadot output; rw_add input
function omegadot = fcn(M, Is, omega,rw_add)
omegadot1=(M(1)-(Is(3,3)-Is(2,2))*omega(2)*omega(3)-rw_add(1))/Is(1,1);
omegadot2=(M(2)-(Is(1,1)-Is(3,3))*omega(1)*omega(3)-rw_add(2))/Is(2,2);
omegadot3=(M(3)-(Is(2,2)-Is(1,1))*omega(1)*omega(2)-rw_add(3))/Is(3,3);
omegadot = [omegadot1 omegadot2 omegadot3];

== matlab function Satellite_Design_Model_2019ver/R//W Dynamics + Gyroscopic Effect ==
  data: Irw input; rw_add output; omega_s input; omega_rw input; omega_rwdot input
function rw_add = fcn(Irw,omega_s,omega_rw,omega_rwdot)
rwx = Irw(1,1)*(omega_rwdot(1)+omega_rw(3)*omega_s(2)-omega_rw(2)*omega_s(3));
rwy = Irw(2,2)*(omega_rwdot(2)+omega_rw(1)*omega_s(3)-omega_rw(3)*omega_s(1));
rwz = Irw(3,3)*(omega_rwdot(3)+omega_rw(2)*omega_s(1)-omega_rw(1)*omega_s(2));
rw_add = [rwx rwy rwz];

== matlab function Satellite_Design_Model_2019ver/Conversion Matrix from Angluar Velocity to Euler Angles ==
  data: omega input; thetadot output; theta input
function thetadot = fcn(omega,theta)
thetadot1=(cos(theta(3))/cos(theta(2)))*omega(1)-(sin(theta(3))/cos(theta(2)))*omega(2);
thetadot2=sin(theta(3))*omega(1)+cos(theta(3))*omega(2);
thetadot3=(-sin(theta(2))*cos(theta(3))/cos(theta(2)))*omega(1)+(sin(theta(2))*sin(theta(3))/cos(theta(2)))*omega(2)+omega(3);
thetadot = [thetadot1 thetadot2 thetadot3];

== matlab function Satellite_Design_Model_2019ver/Inertial to Orbit Rotation Matrix ==
  data: r input; Mo output; ro input; Vo input; Mi input
function Mo = fcn(r,ro,Vo,Mi)
z=-r/norm(r);
H =cross(ro,Vo);
y=-H/norm(H);
x=cross(y,z);
R = [x y z];
Mo = R'*Mi;

== matlab function Satellite_Design_Model_2019ver/Gravity Gradient Moment/Gravity Gradient Matrix ==
  data: r input; Mgg output; I input
function Mgg = fcn(r,I)
miu=3.986E14;
resultantR=((r(1)^2)+(r(2)^2)+(r(3)^2))^(1/2);

%Defining u
ux=r(1)*(-1)/resultantR;
uy=r(2)*(-1)/resultantR;
uz=r(3)*(-1)/resultantR;
u=[ux ; uy ; uz];

%The variables to calculate gravity gradient
firstone=(3*miu/(resultantR^3))*u;
secondone=I*u;

Mgg = cross(firstone,secondone);

== matlab function Satellite_Design_Model_2019ver/Initial Orbital Radius and Velocity ==
  data: Vo output; a input; e input; ro output; i input; u input; RAAN input; theta input
function [Vo,ro] = fcn(a,e,i,u,RAAN,theta)
miu = 3.986E5;
%Rotation matrix converting orbital to inertial
Rio = [-sin(RAAN)*cos(i)*sin(u)+cos(RAAN)*cos(u) -sin(RAAN)*cos(i)*cos(u)-cos(RAAN)*sin(u)...
     sin(RAAN)*sin(i) ;cos(RAAN)*cos(i)*sin(u)+sin(RAAN)*cos(u) cos(RAAN)*cos(i)*cos(u)-sin(RAAN)*sin(u)...
     -cos(RAAN)*sin(i) ;sin(i)*sin(u) sin(i)*cos(u) sin(i)];
%Initial radius and velocity orbital
r = [((a*(1-(e^2)))/(1+(e*cos(theta))))*cos(theta) ;((a*(1-(e^2)))/(1+(e*cos(theta))))*sin(theta) ;0];
V = [-sqrt(miu/(a*(1-e^2)))*sin(theta) ;sqrt(miu/(a*(1-e^2)))*(cos(theta)+e) ;0];


ro = Rio*r;
Vo = Rio*V;

== matlab function Satellite_Design_Model_2019ver/  ==
  data: theta input; Torque output; Be input; moment input
function Torque = fcn(theta,Be,moment)
Torque=zeros(3,1);
Torque=[moment*Be*sin(theta(1));0;moment*Be*sin(theta(3))];

== matlab function Satellite_Design_Model_2019ver/Convert to Euler Angle ==
  data: r input; euler output
function euler = fcn(r)
resultantR=((r(1)^2)+(r(2)^2)+(r(3)^2))^(1/2);

x = -r(1);
y = -r(2);
z = -r(3);

eulerZ = atan(y/x);
eulerY = asin(z/resultantR);
eulerX = 0;

euler = [eulerZ  eulerY  eulerX];

== matlab function Satellite_Design_Model_2019ver/Ephemeris to Euler Satellite/Convert to Euler Angles ==
  data: r input; euler output
function euler = fcn(r)
resultantR=((r(1)^2)+(r(2)^2)+(r(3)^2))^(1/2);

x = r(1);
y = r(2);
z = r(3);

r = resultantR
eulerZ = atan(y/x);
eulerY = asin(z/r);
eulerX = 0;

euler = [eulerZ eulerY eulerX]

%Defining a
% ax = r(1)/resultantR;
% ay = r(2)/resultantR;
% az = r(3)/resultantR;
% psi = 0
% 
% Calculation of Rotation Matrix
% r11 = (ax^2) + (cos(psi)*(1-ax^2));
% r12 = (ax*ay*(1-cos(psi))) + (az*sin(psi));
% r13 = (ax*az*(1-cos(psi))) - (ay*sin(psi));
% r21 = (ax*ay*(1-cos(psi))) - (az*sin(psi));
% r22 = (ay^2) + (cos(psi)*(1-ay^2));
% r23 = (ay*az*(1-cos(psi))) + (ax*sin(psi));
% r31 = (ax*az*(1-cos(psi))) + (ay*sin(psi));
% r32 = (ay*az*(1-cos(psi))) - (ax*sin(psi));
% r33 = (az^2) + (cos(psi)*(1-az^2));
% RotationMatrix = [r11 r12 r13;r21 r22 r23;r31 r32 r33];
% 
% RotationMatrix = RotationMatrix;
